simulink model "main041_Decouple"  (R2023b)
settings: Solver=VariableStepAuto  StartTime=0.0  StopTime=10.0  RelTol=1e-3
settings Model: Creator=YYlab_05  LastModifiedBy=YYlab_05

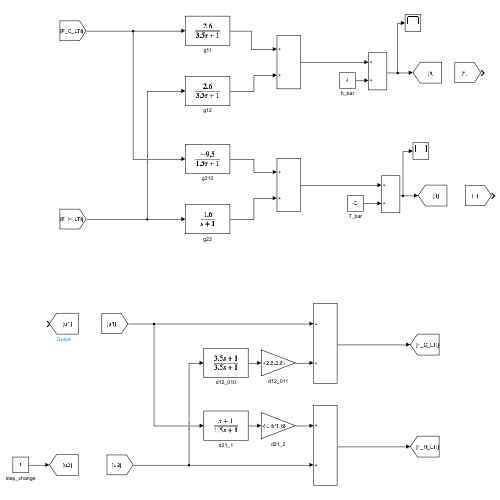
[thumbnail: Simulink's stored preview of the top-level diagram]
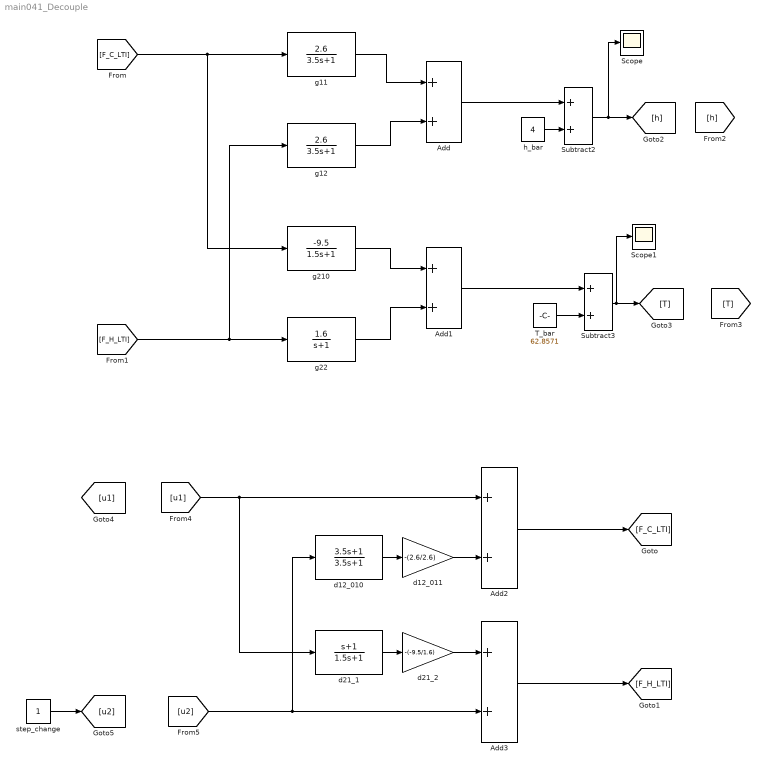
== system main041_Decouple ==
  Add{,1..3} (4 alike) : Sum
  Scope : Scope
  Scope1 : Scope
  Subtract2 : Sum
  Subtract3 : Sum
  T_bar : Constant  Value=62.8571
  d12_010 : TransferFcn  Numerator=[3.5 1]  Denominator=[3.5 1]
  d12_011 : Gain  Gain=-(2.6/2.6)
  d21_1 : TransferFcn  Numerator=[1 1]  Denominator=[1.5 1]
  d21_2 : Gain  Gain=-(-9.5/1.6)
  g11 : TransferFcn  Numerator=[2.6]  Denominator=[3.5 1]
  g12 : TransferFcn  Numerator=2.6  Denominator=[3.5 1]
  g210 : TransferFcn  Numerator=[-9.5]  Denominator=[1.5 1]
  g22 : TransferFcn  Numerator=1.6  Denominator=[1 1]
  h_bar : Constant  Value=4
  step_change : Constant
  wires:
  [F_C_LTI] -> g11/1, g210/1
  [F_H_LTI] -> g22/1, g12/1
  g11/1 -> Add/1
  Add/1 -> Subtract2/1
  g22/1 -> Add1/2
  g12/1 -> Add/2
  g210/1 -> Add1/1
  Add2/1 -> [F_C_LTI]
  Add3/1 -> [F_H_LTI]
  h_bar/1 -> Subtract2/2
  Subtract2/1 -> Scope/1, [h]
  T_bar/1 -> Subtract3/2
  Add1/1 -> Subtract3/1
  Subtract3/1 -> Scope1/1, [T]
  [u2] -> Add3/2, d12_010/1
  d12_010/1 -> d12_011/1
  d12_011/1 -> Add2/2
  [u1] -> Add2/1, d21_1/1
  d21_1/1 -> d21_2/1
  d21_2/1 -> Add3/1
  step_change/1 -> [u2]
